simulink model "Z_CL1"  (R2024a)
settings: Solver=FixedStepDiscrete  StartTime=0.0  StopTime=inf  FixedStep=Tsw  RelTol=1e-3  EnableMultiTasking=on
undefined symbols (not defined in the file or in its folder): ADC_mapping, DiscIntNeverNeededParam, Down, IfbMax, ILmax, kaw_i, kaw_v, ki_i, ki_v, kp_i, kp_v, Rload, TBPRD, Tsw, Up, VfbMax, VinNom, VLlim, VoutMax, zden_aaf, zden_plant_i, zden_plant_v, znum_aaf, znum_plant_i, znum_plant_v
libraries: c280xlib x4, simulink x1, demo_controls x1, svdschedulerlib x1
settings Model: Creator=The MathWorks, Inc.  LastModifiedBy=nicholas
settings SolverCC: AlgebraicLoopSolver=TrustRegion
settings DataIOCC: LimitDataPoints=on  SaveFormat=Array  SaveOutput=off  SaveTime=off  ReturnWorkspaceOutputs=off
settings OptimizationCC: ExpressionDepthLimit=2147483647  InitFltsAndDblsToZero=on  LifeSpan=inf  MaxStackSize=64
settings DebuggingCC: UnderspecifiedInitializationDetection=Classic  MergeDetectMultiDrivingBlocksExec=none  SignalResolutionControl=TryResolveAllWithWarning  InheritedTsInSrcMsg=none  MultiTaskDSMMsg=warning  MultiTaskCondExecSysMsg=none  FcnCallInpInsideContextMsg=warning  UnconnectedInputMsg=warning  UnconnectedOutputMsg=warning  UnconnectedLineMsg=warning  AllowSymbolicDim=off  StateNameClashWarn=warning  SFUnexpectedBacktrackingDiag=warning  SFNoUnconditionalDefaultTransitionDiag=warning  SFExecutionAtInitializationDiag=none  ArithmeticOperatorsInVariantConditions=warning
settings HardwareCC: ProdBitPerChar=16  ProdBitPerInt=16  ProdBitPerPointer=32  ProdBitPerSizeT=32  ProdBitPerPtrDiffT=32  ProdLargestAtomicInteger=Integer  ProdLargestAtomicFloat=None  ProdWordSize=16  ProdHWDeviceType=Texas Instruments->C2000  TargetBitPerChar=16  TargetBitPerInt=16  TargetBitPerPointer=16  TargetLargestAtomicInteger=Integer  TargetIntDivRoundTo=Zero  TargetEndianess=LittleEndian  TargetWordSize=16  TargetHWDeviceType=Texas Instruments->C2000  ProdEqTarget=off  UseEmbeddedCoderFeatures=off
settings ModelReferenceCC: EnableRefExpFcnMdlSchedulingChecks=on  PropagateSignalLabelsOutOfModel=off
settings SFSimCC: SimUseLocalCustomCode=off  MATLABDynamicMemAlloc=off  CustomCodeUndefinedFunction=UseInterfaceOnly
settings RTWCC: Description=Embedded Coder  SystemTargetFile=ert.tlc  HardwareBoard=TI Delfino F2833x  TemplateMakefile=ert_default_tmf  PostCodeGenCommand=; codertarget.postCodeGenHookCommand(h)  RTWUseLocalCustomCode=off  Toolchain=Texas Instruments Code Composer Studio (C2000)  GPUComputeCapability=3.5
settings CodeAppCC: StateflowObjectComments=on
settings ERTTargetCC: MultiwordLength=2048  ParMdlRefBuildCompliant=off  CompOptLevelCompliant=off  ConcurrentExecutionCompliant=off  ERTCustomFileBanners=off  SupportContinuousTime=on  SupportNonInlinedSFcns=on  RemoveResetFunc=off  ModelStepFunctionPrototypeControlCompliant=off  CPPClassGenCompliant=off  ExtModeStaticAllocSize=2048  ExtModeMexFile=TIC2000ExternalModeOpen  ExtModeIntrfLevel=Level2 - Open  ConvertIfToSwitch=off  SuppressUnreachableDefaultCases=off
settings ConfigComp: CovMetricSettings=dw  CovSaveCumulativeToWorkspaceVar=on  CovSaveSingleToWorkspaceVar=on  CovExternalEMLEnable=off  CovSFcnEnable=off

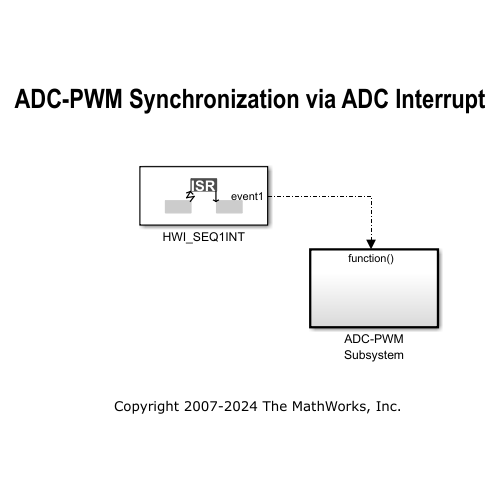
[thumbnail: Simulink's stored preview of the top-level diagram]
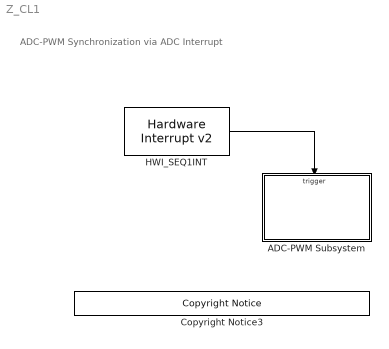
== system Z_CL1 ==
  note: ADC-PWM Synchronization via ADC Interrupt
  ADC-PWM Subsystem : Subsystem  TreatAsAtomicUnit=on
  Copyright Notice3 : demo_controls/Copyright Notice  year=2007  prod=tic2000
  HWI_SEQ1INT : svdschedulerlib/Hardware Interrupt v2  ISRGroup=ADC - Analog to Digital Converter  ISRName=ADCA1_INT  ISRNumber=32  NumEventsToServe=1  EventsList={'on','EOC event','1';'off','Overflow event','2';'off','Custom event','3'}  SelectedEvents={'event1'}  TaskPriority=30  DisablePreemption=on  ClearInterruptFlagsAtEndOfEvent=on  InterruptDefinitionFile=$(TARGET_ROOT)/registry/interrupts/F2837xS_interrupts.xml  HardwareBoard=F2837x  EnableSimPort=off
      settings: LibrarySourceBlock=c2000lib/Scheduling/Hardware Interrupt
  wires:
  HWI_SEQ1INT/1 -> ADC-PWM Subsystem/Trigger

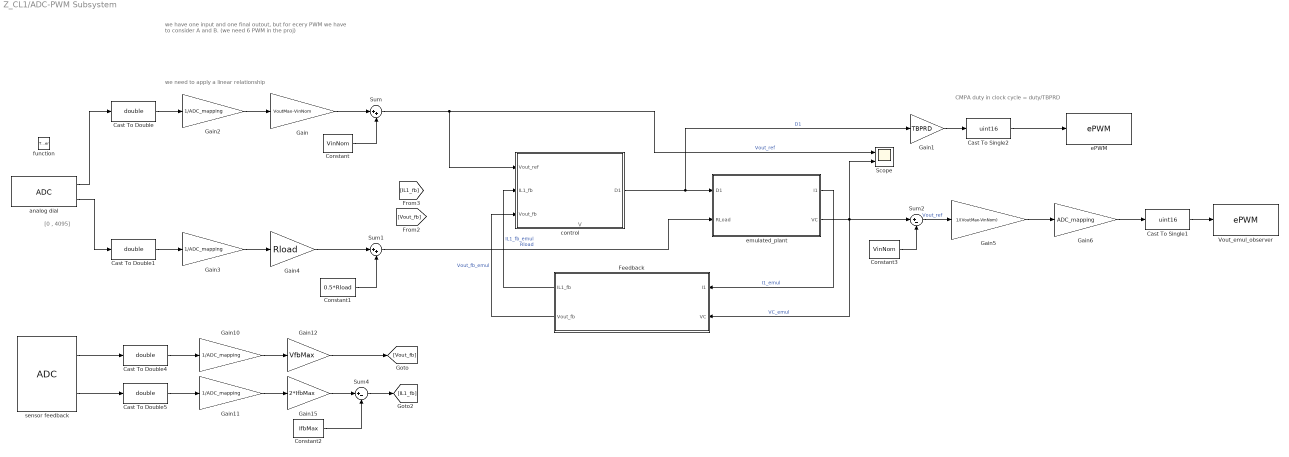
== system Z_CL1/ADC-PWM Subsystem ==
  note: CMPA duty in clock cycle = duty/TBPRD
  note: V
  note: we need to apply a linear relationship
  note: we have one input and one final outout, but for ecery PWM we
      | have to consider A and B. (we need 6 PWM in the proj)
  note: [0 , 4095]
  function : TriggerPort  TriggerType=function-call  VariantControl=Variant
  Cast To Double{,1,4..5} (4 alike) : DataTypeConversion  OutDataTypeStr=double  SaturateOnIntegerOverflow=off  RndMeth=Floor
  Cast To Single1 : DataTypeConversion  OutDataTypeStr=uint16  SaturateOnIntegerOverflow=off  RndMeth=Floor
  Cast To Single2 : DataTypeConversion  OutDataTypeStr=uint16  SaturateOnIntegerOverflow=off  RndMeth=Floor
  Constant : Constant  Value=VinNom
  Constant1 : Constant  Value=0.5*Rload
  Constant2 : Constant  Value=IfbMax
  Constant3 : Constant  Value=VinNom
  Feedback : Subsystem
  Gain : Gain  Gain=VoutMax-VinNom
  Gain1 : Gain  Gain=TBPRD
  Gain{2..3,10..11} (4 alike) : Gain  Gain=1/ADC_mapping
  Gain12 : Gain  Gain=VfbMax
  Gain15 : Gain  Gain=2*IfbMax
  Gain4 : Gain  Gain=Rload
  Gain5 : Gain  Gain=1/(VoutMax-VinNom)
  Gain6 : Gain  Gain=ADC_mapping
  Scope : Scope  NumInputPorts=2
  Sum : Sum  Inputs=|++
  Sum1 : Sum  Inputs=|++
  Sum2 : Sum  Inputs=|+-
  Sum4 : Sum  Inputs=|+-
  Vout_emul_observer : c280xlib/ePWM  checkMode=off  useModule=ePWM1  periodUnits=Clock cycles  timerSource=Specify via dialog  timerPeriod_clk=TBPRD  timerPeriod_sec=0.0001  tbshadow=Counter equals to zero  countingMode=Up-Down  phaseActiveEnable=Disable  phaseDirection=Count down after sync  phaseActive=TBPRD*2/3  synchronizationEnable=off  synchronizationOption=Counter equals to zero (CTR=Zero)  clockPrescale=1  HSclockPrescale=1  ePWMxAStatus=off  CMPAUnits=Clock cycles  CMPASource=Input port  CMPAValue_per=50  CMPAValue_clk=0  enCMPAshadow=Counter equals to zero  ePWMxAactionLogic1=Do nothing  ePWMxAactionLogic2=Do nothing  ePWMxAactionLogic3=Set  ePWMxAactionLogic4=Clear  ePWMxAactionLogic5=Do nothing  ePWMxAactionLogic6=Do nothing  ePWMxALoadMode=Load on counter equals to zero (CTR=Zero)  ePWMxACSFenable=off  ePWMxACSFvalue=Forcing disable  ePWMxASFreload=Zero  enHRPWM=off  HRPWM_LoadMode=Counter equals to zero (CTR=ZERO)  HRPWM_CTLMode=Phase control mode  HRPWM_EDGMode=Both edge  enSFO=on  ePWMxBStatus=off  CMPBUnits=Clock cycles  CMPBSource=Specify via dialog  CMPBValue_per=0  CMPBValue_clk=0  enCMPBshadow=Counter equals to zero  ePWMxBactionLogic1=Do nothing  ePWMxBactionLogic2=Set  ePWMxBactionLogic3=Do nothing  ePWMxBactionLogic4=Do nothing  ePWMxBactionLogic5=Clear  ePWMxBactionLogic6=Do nothing  ePWMxBLoadMode=Load on counter equals to zero (CTR=Zero)  ePWMxBCSFenable=off  ePWMxBCSFvalue=Forcing disable  ePWMxBSFreload=Zero  enableDBePWMxA=off  enableDBePWMxB=off  DBpolarity=Active high complementary (AHC)  DBedgeDelay=Positive  DBSource_ePWMxA=ePWMxA  DBSource_ePWMxB=ePWMxA  DBperiodSource=Specify via dialog  REDperiod=DBFED  FEDperiod=DBFED  adcstartModuleA=off  adcrequestEventA=First event  adcstartEventA=Counter equals to period (CTR=PRD)  adcstartModuleB=off  adcrequestEventB=First event  adcstartEventB=Counter equals to zero (CTR=Zero)  intEn=off  intPrd=First event  intSel=Counter equals to zero (CTR=Zero)  chopperEnable=off  chopperFrequency=1  chopperFirstwidth=1  chopperDuty=12.5%  tripZonesource=Specify via dialog  tzselOSHT1=off  tzselOSHT2=off  tzselOSHT3=off  tzselOSHT4=off  tzselOSHT5=off  tzselOSHT6=off  tzselCBC1=off  tzselCBC2=off  tzselCBC3=off  tzselCBC4=off  tzselCBC5=off  tzselCBC6=off  enTzOstIntr=off  enTzCbcIntr=off  ePWMxAforced=No action  ePWMxBforced=No action  timerPeriod=-1  ePWMxAValue=1  ePWMxBValue=0  tripZoneoption=One-shot trip (OSHT)
  analog dial : c280xlib/ADC  useModule=A  useMode=Sequential  sourceSOC=Software  sourceSOC1=ePWMxA  sourceSOC2=ePWMxB  xint2_ADCSOC=31  Ts=-1  dType=double  postInterrupt=on  endma=off  chdma=1  numConversionsSingle=2  numConversionsDouble=1  conv0=ADCINA0  conv1=ADCINA1  conv2=ADCINA2  conv3=ADCINA3  conv4=ADCINA4  conv5=ADCINA5  conv6=ADCINA6  conv7=ADCINA7  conv8=ADCINB0  conv9=ADCINB1  conv10=ADCINB2  conv11=ADCINB3  conv12=ADCINB4  conv13=ADCINB5  conv14=ADCINB6  conv15=ADCINB7  convAB0=ADCINA0 and ADCINB0  convAB1=ADCINA1 and ADCINB1  convAB2=ADCINA2 and ADCINB2  convAB3=ADCINA3 and ADCINB3  convAB4=ADCINA4 and ADCINB4  convAB5=ADCINA5 and ADCINB5  convAB6=ADCINA6 and ADCINB6  convAB7=ADCINA7 and ADCINB7  convA0=ADCINA0  convA1=ADCINA1  convA2=ADCINA2  convA3=ADCINA3  convA4=ADCINA4  convA5=ADCINA5  convA6=ADCINA6  convA7=ADCINA7  convB0=ADCINB0  convB1=ADCINB1  convB2=ADCINB2  convB3=ADCINB3  convB4=ADCINB4  convB5=ADCINB5  convB6=ADCINB6  convB7=ADCINB7  c28xmultiPort=on
  control : Subsystem
  ePWM : c280xlib/ePWM  checkMode=off  useModule=ePWM2  periodUnits=Clock cycles  timerSource=Specify via dialog  timerPeriod_clk=TBPRD  timerPeriod_sec=0.0001  tbshadow=Counter equals to zero  countingMode=Up-Down  phaseActiveEnable=Set counter to phase value specified via dialog  phaseDirection=Count down after sync  phaseActive=0  synchronizationEnable=off  synchronizationOption=Counter equals to zero (CTR=Zero)  clockPrescale=1  HSclockPrescale=1  ePWMxAStatus=on  CMPAUnits=Clock cycles  CMPASource=Input port  CMPAValue_per=50  CMPAValue_clk=0  enCMPAshadow=Counter equals to zero  ePWMxAactionLogic1=Do nothing  ePWMxAactionLogic2=Do nothing  ePWMxAactionLogic3=Set  ePWMxAactionLogic4=Clear  ePWMxAactionLogic5=Do nothing  ePWMxAactionLogic6=Do nothing  ePWMxALoadMode=Load on counter equals to zero (CTR=Zero)  ePWMxACSFenable=off  ePWMxACSFvalue=Forcing disable  ePWMxASFreload=Zero  enHRPWM=off  HRPWM_LoadMode=Counter equals to zero (CTR=ZERO)  HRPWM_CTLMode=Phase control mode  HRPWM_EDGMode=Both edge  enSFO=on  ePWMxBStatus=off  CMPBUnits=Clock cycles  CMPBSource=Specify via dialog  CMPBValue_per=0  CMPBValue_clk=0  enCMPBshadow=Counter equals to zero  ePWMxBactionLogic1=Do nothing  ePWMxBactionLogic2=Set  ePWMxBactionLogic3=Do nothing  ePWMxBactionLogic4=Do nothing  ePWMxBactionLogic5=Clear  ePWMxBactionLogic6=Do nothing  ePWMxBLoadMode=Load on counter equals to zero (CTR=Zero)  ePWMxBCSFenable=off  ePWMxBCSFvalue=Forcing disable  ePWMxBSFreload=Zero  enableDBePWMxA=on  enableDBePWMxB=on  DBpolarity=Active high complementary (AHC)  DBedgeDelay=Positive  DBSource_ePWMxA=ePWMxA  DBSource_ePWMxB=ePWMxA  DBperiodSource=Specify via dialog  REDperiod=DBFED  FEDperiod=DBFED  adcstartModuleA=on  adcrequestEventA=First event  adcstartEventA=Counter equals to period (CTR=PRD)  adcstartModuleB=off  adcrequestEventB=First event  adcstartEventB=Counter equals to zero (CTR=Zero)  intEn=off  intPrd=First event  intSel=Counter is incrementing and equals to the compare A register (CTRU=CMPA)  chopperEnable=off  chopperFrequency=1  chopperFirstwidth=1  chopperDuty=12.5%  tripZonesource=Specify via dialog  tzselOSHT1=off  tzselOSHT2=off  tzselOSHT3=off  tzselOSHT4=off  tzselOSHT5=off  tzselOSHT6=off  tzselCBC1=off  tzselCBC2=off  tzselCBC3=off  tzselCBC4=off  tzselCBC5=off  tzselCBC6=off  enTzOstIntr=off  enTzCbcIntr=off  ePWMxAforced=No action  ePWMxBforced=No action  timerPeriod=-1  ePWMxAValue=1  ePWMxBValue=0  tripZoneoption=One-shot trip (OSHT)
  emulated_plant : Subsystem
  sensor feedback : c280xlib/ADC  useModule=A  useMode=Sequential  sourceSOC=Software  sourceSOC1=ePWMxA  sourceSOC2=ePWMxB  xint2_ADCSOC=31  Ts=-1  dType=double  postInterrupt=on  endma=off  chdma=1  numConversionsSingle=2  numConversionsDouble=1  conv0=ADCINA0  conv1=ADCINA1  conv2=ADCINA2  conv3=ADCINA3  conv4=ADCINA4  conv5=ADCINA5  conv6=ADCINA6  conv7=ADCINA7  conv8=ADCINB0  conv9=ADCINB1  conv10=ADCINB2  conv11=ADCINB3  conv12=ADCINB4  conv13=ADCINB5  conv14=ADCINB6  conv15=ADCINB7  convAB0=ADCINA0 and ADCINB0  convAB1=ADCINA1 and ADCINB1  convAB2=ADCINA2 and ADCINB2  convAB3=ADCINA3 and ADCINB3  convAB4=ADCINA4 and ADCINB4  convAB5=ADCINA5 and ADCINB5  convAB6=ADCINA6 and ADCINB6  convAB7=ADCINA7 and ADCINB7  convA0=ADCINA4  convA1=ADCINA5  convA2=ADCINA4  convA3=ADCINA5  convA4=ADCINA4  convA5=ADCINA5  convA6=ADCINA6  convA7=ADCINA7  convB0=ADCINB0  convB1=ADCINB1  convB2=ADCINB2  convB3=ADCINB3  convB4=ADCINB4  convB5=ADCINB5  convB6=ADCINB6  convB7=ADCINB7  c28xmultiPort=on
  wires:
  Gain1/1 -> Cast To Single2/1
  Cast To Single2/1 -> ePWM/1
  Feedback/1(IL1_fb) -> control/2(IL1_fb)  "IL1_fb_emul"
  Feedback/2(Vout_fb) -> control/3(Vout_fb)  "Vout_fb_emul"
  emulated_plant/1(I1) -> Feedback/1(I1)  "I1_emul"
  Constant2/1 -> Sum4/2
  Sum1/1 -> emulated_plant/2(RLoad)  "Rload"
  analog dial/2 -> Cast To Double1/1
  Sum/1 -> Scope/1, control/1(Vout_ref)  "Vout_ref"
  Constant/1 -> Sum/2
  control/1(D1) -> Gain1/1, emulated_plant/1(D1)  "D1"
  Gain4/1 -> Sum1/1
  Gain/1 -> Sum/1
  Cast To Double/1 -> Gain2/1
  analog dial/1 -> Cast To Double/1
  Gain5/1 -> Gain6/1
  Constant1/1 -> Sum1/2
  Sum4/1 -> [IL1_fb]
  Cast To Double5/1 -> Gain11/1
  emulated_plant/2(VC) -> Sum2/1, Scope/2, Feedback/2(VC)  "VC_emul"
  Gain10/1 -> Gain12/1
  Cast To Double1/1 -> Gain3/1
  Gain2/1 -> Gain/1
  Cast To Double4/1 -> Gain10/1
  Gain15/1 -> Sum4/1
  Cast To Single1/1 -> Vout_emul_observer/1
  sensor feedback/2 -> Cast To Double5/1
  Gain12/1 -> [Vout_fb]
  Gain3/1 -> Gain4/1
  sensor feedback/1 -> Cast To Double4/1
  Gain11/1 -> Gain15/1
  Sum2/1 -> Gain5/1  "Vout_ref"
  Constant3/1 -> Sum2/2
  Gain6/1 -> Cast To Single1/1

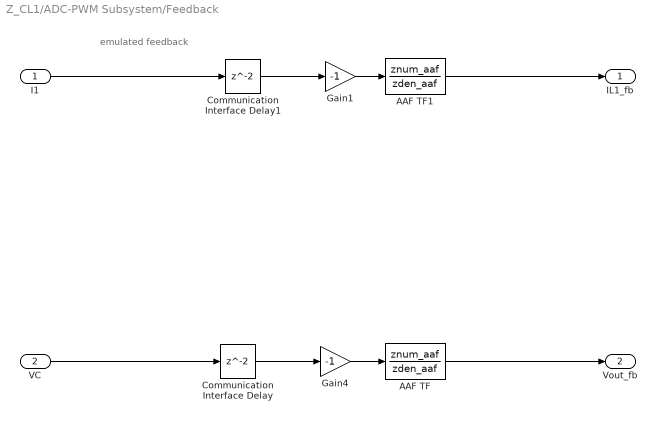
== system Z_CL1/ADC-PWM Subsystem/Feedback ==
  note: emulated feedback
  I1 : Inport
  VC : Inport  Port=2
  AAF TF : DiscreteTransferFcn  Numerator=znum_aaf  Denominator=zden_aaf
  AAF TF1 : DiscreteTransferFcn  Numerator=znum_aaf  Denominator=zden_aaf
  Communication Interface Delay : Delay
  Communication Interface Delay1 : Delay
  Gain1 : Gain  Gain=-1
  Gain4 : Gain  Gain=-1
  IL1_fb : Outport
  Vout_fb : Outport  Port=2
  wires:
  I1/1 -> Communication Interface Delay1/1
  AAF TF/1 -> Vout_fb/1
  Gain1/1 -> AAF TF1/1
  AAF TF1/1 -> IL1_fb/1
  Communication Interface Delay1/1 -> Gain1/1
  Communication Interface Delay/1 -> Gain4/1
  VC/1 -> Communication Interface Delay/1
  Gain4/1 -> AAF TF/1

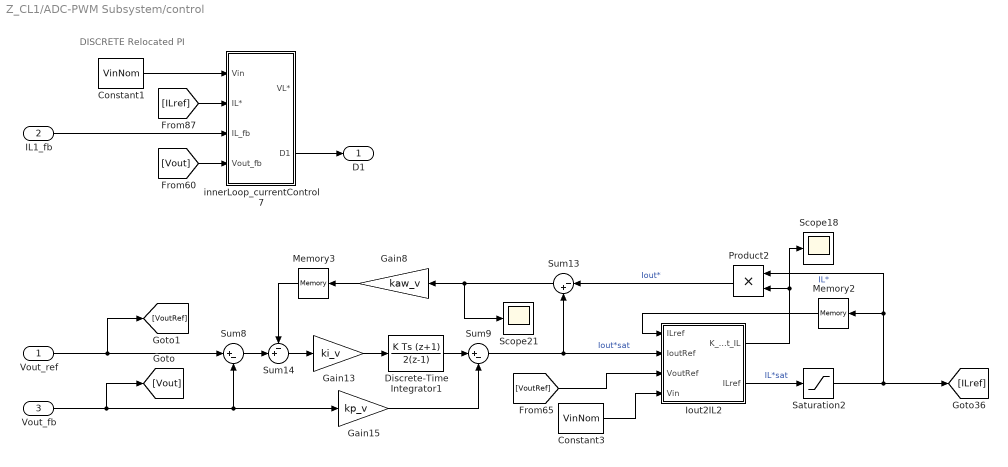
== system Z_CL1/ADC-PWM Subsystem/control ==
  note: DISCRETE Relocated PI
  Vout_ref : Inport
  IL1_fb : Inport  Port=2
  Vout_fb : Inport  Port=3
  Constant1 : Constant  Value=VinNom
  Constant3 : Constant  Value=VinNom
  Discrete-Time Integrator1 : DiscreteIntegrator  IntegratorMethod=Integration: Trapezoidal  SampleTime=Tsw  ICPrevOutput=DiscIntNeverNeededParam  ICPrevScaledInput=DiscIntNeverNeededParam
  Gain13 : Gain  Gain=ki_v
  Gain15 : Gain  Gain=kp_v
  Gain8 : Gain  Gain=kaw_v
  Iout2IL2 : MATLAB Function  TreatAsAtomicUnit=on
  Memory2 : Memory
  Memory3 : Memory
  Product2 : Product
  Saturation2 : Saturate  UpperLimit=ILmax  LowerLimit=-ILmax
  Scope18 : Scope
  Scope21 : Scope
  Sum13 : Sum  Inputs=|-+
  Sum14 : Sum  Inputs=-+|
  Sum8 : Sum  Inputs=|+-
  Sum9 : Sum  Inputs=|+-
  innerLoop_currentControl7 : Subsystem
  D1 : Outport
  wires:
  Vout_fb/1 -> [Vout], Gain15/1, Sum8/2
  Vout_ref/1 -> [VoutRef], Sum8/1
  [VoutRef] -> Iout2IL2/3(VoutRef)
  Constant1/1 -> innerLoop_currentControl7/1(Vin)
  Iout2IL2/1(K_Iout_IL) -> Product2/2, Scope18/1
  Gain8/1 -> Memory3/1
  IL1_fb/1 -> innerLoop_currentControl7/3(IL_fb)
  Sum9/1 -> Sum13/2, Iout2IL2/2(IoutRef)  "Iout*sat"
  innerLoop_currentControl7/2(D1) -> D1/1
  [ILref] -> innerLoop_currentControl7/2(IL*)
  Memory2/1 -> Iout2IL2/1("ILref ")
  Sum13/1 -> Scope21/1, Gain8/1
  Memory3/1 -> Sum14/1
  Iout2IL2/2(ILref) -> Saturation2/1  "IL*sat"
  [Vout] -> innerLoop_currentControl7/4(Vout_fb)
  Sum14/1 -> Gain13/1
  Sum8/1 -> Sum14/2
  Gain15/1 -> Sum9/2
  Gain13/1 -> Discrete-Time Integrator1/1
  Discrete-Time Integrator1/1 -> Sum9/1
  Saturation2/1 -> [ILref], Product2/1, Memory2/1  "IL*"
  Product2/1 -> Sum13/1  "Iout*"
  Constant3/1 -> Iout2IL2/4(Vin)

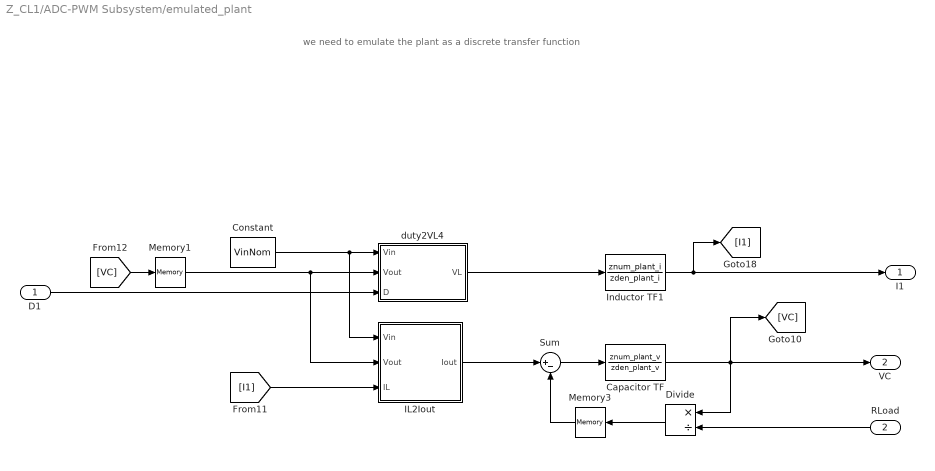
== system Z_CL1/ADC-PWM Subsystem/emulated_plant ==
  note: we need to emulate the plant as a discrete transfer function
  D1 : Inport
  RLoad : Inport  Port=2
  Capacitor TF : DiscreteTransferFcn  Numerator=znum_plant_v  Denominator=zden_plant_v
  Constant : Constant  Value=VinNom
  Divide : Product  Inputs=*/
  IL2Iout : MATLAB Function  TreatAsAtomicUnit=on
  Inductor TF1 : DiscreteTransferFcn  Numerator=znum_plant_i  Denominator=zden_plant_i
  Memory1 : Memory
  Memory3 : Memory
  Sum : Sum  Inputs=|+-
  duty2VL4 : MATLAB Function  TreatAsAtomicUnit=on
  I1 : Outport
  VC : Outport  Port=2
  wires:
  Capacitor TF/1 -> VC/1, [VC], Divide/1
  Divide/1 -> Memory3/1
  [I1] -> IL2Iout/3(IL)
  RLoad/1 -> Divide/2
  D1/1 -> duty2VL4/3(D)
  Inductor TF1/1 -> [I1], I1/1
  Constant/1 -> IL2Iout/1(Vin), duty2VL4/1(Vin)
  Sum/1 -> Capacitor TF/1
  [VC] -> Memory1/1
  duty2VL4/1(VL) -> Inductor TF1/1
  IL2Iout/1(Iout) -> Sum/1
  Memory3/1 -> Sum/2
  Memory1/1 -> IL2Iout/2(Vout), duty2VL4/2(Vout)

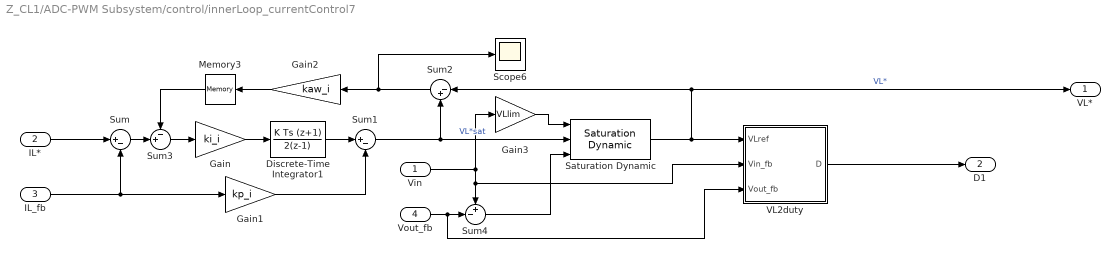
== system Z_CL1/ADC-PWM Subsystem/control/innerLoop_currentControl7 ==
  Vin : Inport
  IL* : Inport  Port=2
  IL_fb : Inport  Port=3
  Vout_fb : Inport  Port=4
  Discrete-Time Integrator1 : DiscreteIntegrator  IntegratorMethod=Integration: Trapezoidal  SampleTime=Tsw  ICPrevOutput=DiscIntNeverNeededParam  ICPrevScaledInput=DiscIntNeverNeededParam
  Gain : Gain  Gain=ki_i
  Gain1 : Gain  Gain=kp_i
  Gain2 : Gain  Gain=kaw_i
  Gain3 : Gain  Gain=VLlim
  Memory3 : Memory
  Saturation Dynamic : simulink/Discontinuities/Saturation Dynamic  OutMin=[]  OutMax=[]  OutDataTypeStr=Inherit: Same as second input  OutDataType=fixdt(1, 16)  OutScaling=2^-10  DoSatur=off
  Scope6 : Scope
  Sum : Sum  Inputs=|+-
  Sum1 : Sum  Inputs=|+-
  Sum2 : Sum  Inputs=|-+
  Sum3 : Sum  Inputs=-+|
  Sum4 : Sum  Inputs=+-|
  VL2duty : MATLAB Function  TreatAsAtomicUnit=on
  VL* : Outport
  D1 : Outport  Port=2
  wires:
  VL2duty/1(D) -> D1/1
  Sum/1 -> Sum3/2
  Gain3/1 -> Saturation Dynamic/1
  Gain1/1 -> Sum1/2
  Sum3/1 -> Gain/1
  Gain/1 -> Discrete-Time Integrator1/1
  Gain2/1 -> Memory3/1
  Vin/1 -> VL2duty/2(Vin_fb), Sum4/1, Gain3/1
  Sum1/1 -> Saturation Dynamic/2, Sum2/2  "VL*sat"
  Sum4/1 -> Saturation Dynamic/3
  Sum2/1 -> Gain2/1, Scope6/1
  Saturation Dynamic/1 -> VL2duty/1(VLref), VL*/1, Sum2/1  "VL*"
  IL_fb/1 -> Sum/2, Gain1/1
  Vout_fb/1 -> VL2duty/3(Vout_fb), Sum4/2
  Discrete-Time Integrator1/1 -> Sum1/1
  IL*/1 -> Sum/1
  Memory3/1 -> Sum3/1

== matlab function Z_CL1/ADC-PWM Subsystem/emulated_plant/duty2VL4 ==
  data: Vin input; Vout input; D input; VL output
function VL = fcn(Vin,Vout,D)

VL = min((D-1)*Vout + Vin, Vin);

== matlab function Z_CL1/ADC-PWM Subsystem/control/Iout2IL2 ==
  data: K_Iout_IL output; ILref input; IoutRef input; VoutRef input; Vin input; ILref output; RserL parameter
function [K_Iout_IL,ILref] = fcn(ILref,IoutRef,VoutRef,Vin,RserL)

if VoutRef < Vin
    VoutRef = Vin;
end
K_Iout_IL = (Vin - RserL*ILref) / VoutRef;
ILref = IoutRef / K_Iout_IL;

== matlab function Z_CL1/ADC-PWM Subsystem/emulated_plant/IL2Iout ==
  data: Vin input; Vout input; Iout output; IL input; RserL parameter
function Iout = fcn(Vin,Vout,IL,RserL)

if Vout < Vin
    Vout = Vin;
end
K_Iout_IL = (Vin - RserL*IL) / Vout;
Iout = IL*K_Iout_IL;

== matlab function Z_CL1/ADC-PWM Subsystem/control/innerLoop_currentControl7/VL2duty ==
  data: VLref input; D output; Vin_fb input; Vout_fb input
function D = fcn(VLref,Vin_fb,Vout_fb)

D = min([1 max([0 1 + (VLref - Vin_fb)/Vout_fb])]);
